simulink model "nonlinear_model"  (R2025a)
settings: Solver=ode45  StartTime=0.0  StopTime=2  FixedStep=0.0001  RelTol=1e-3
model workspace: external: MATLAB File C:\Users\Artur\Documents\Projekt Aktorik und Mechatronik\Implementation_D.m (data not in the file)
values from neighbouring files (symbols this model uses):
  D = 0.5    [Friction_line_identification.m]    (also in Linear_model.m = 0.2; TVRegDiff.m = spdiags( [ -c c ], [ 0 1 ], n, n ) / dx; electromagnetic_actuator.m; nonlinear_model.m)
  F_R = 1    [Friction_line_identification.m]    (also in electromagnetic_actuator.m; nonlinear_model.m)
  K = 3    [Friction_line_identification.m]    (also in Linear_model.m = 2; electromagnetic_actuator.m; nonlinear_model.m)
  M = 100    [Friction_line_identification.m]    (also in electromagnetic_actuator.m; nonlinear_model.m)
  m = 0.5    [Friction_line_identification.m]    (also in Linear_model.m; electromagnetic_actuator.m; nonlinear_model.m)
  Ts = 0.001    [Friction_line_identification.m]    (also in Linear_model.m; electromagnetic_actuator.m; nonlinear_model.m)
  x0 = [0 ; 0]    [Friction_line_identification.m]    (also in Linear_model.m; electromagnetic_actuator.m; nonlinear_model.m)
libraries: simulink x1
settings Model: Creator=Artur  LastModifiedBy=phill

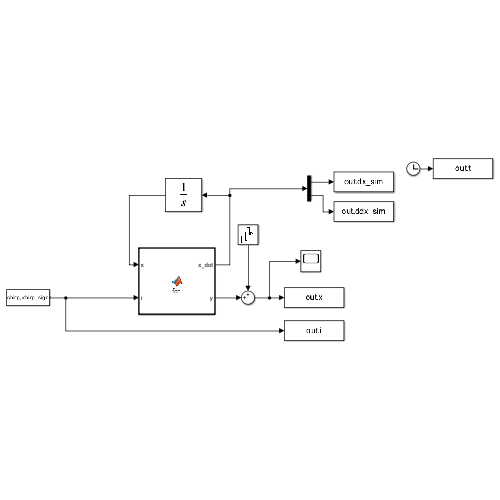
[thumbnail: Simulink's stored preview of the top-level diagram]
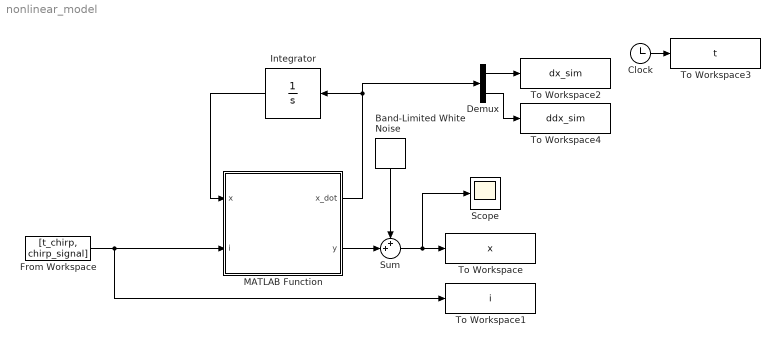
== system nonlinear_model ==
  Band-Limited White Noise : simulink/Sources/Band-Limited White Noise  Cov=[0.00000000001]  Ts=Ts  seed=[23341]
  Clock : Clock
  Demux : Demux  Outputs=2
  From Workspace : FromWorkspace  VariableName=[t_chirp, chirp_signal]
  Integrator : Integrator  InitialCondition=x0
  MATLAB Function : MATLAB Function  TreatAsAtomicUnit=on
  Scope : Scope
      settings: ActiveDisplayYMinimum=-0.05577  ActiveDisplayYMaximum=0.06313
  Sum : Sum  Inputs=++|
  To Workspace : ToWorkspace  VariableName=x  SampleTime=Ts
  To Workspace1 : ToWorkspace  VariableName=i  SampleTime=Ts
  To Workspace2 : ToWorkspace  VariableName=dx_sim  SampleTime=Ts
  To Workspace3 : ToWorkspace  VariableName=t  SampleTime=Ts
  To Workspace4 : ToWorkspace  VariableName=ddx_sim  SampleTime=Ts
  wires:
  From Workspace/1 -> To Workspace1/1, MATLAB Function/2(i)
  Integrator/1 -> MATLAB Function/1(x)
  Clock/1 -> To Workspace3/1
  MATLAB Function/1(x_dot) -> Demux/1, Integrator/1
  Demux/1 -> To Workspace2/1
  Demux/2 -> To Workspace4/1
  Sum/1 -> Scope/1, To Workspace/1
  MATLAB Function/2(y) -> Sum/2
  Band-Limited White Noise/1 -> Sum/1

== matlab function nonlinear_model/MATLAB Function ==
  data: x_dot output; x input; y output; i input; m parameter; M parameter; D parameter; K parameter; F_R parameter
function [x_dot,y] = fcn(x,i,m, M, D, K, F_R)
%% ZRM Linearaktor

x_dot = [x(2);
         (K/m)*i-(D/m)*x(2)-(F_R/m)*atan(M*x(2))];

y = x(1);
end
